simulink model "Q6"  (R2023b)
settings: Solver=VariableStepAuto  StartTime=0.0  StopTime=50  RelTol=1e-3
values from neighbouring files (symbols this model uses):
  A = [ -8.8487+(a-b)/5,           -0.0399,                     -5.55+(c+d)/10,               3.5846 ... (first row only)    [EE5101_Q1 copy.m]    (also in EE5101_Q1.m; Q3.m; Q3_reduced_order.m; Q6.m)
  B = [0.0564+b/(10+c),                       0.0319 ... (first row only)    [EE5101_Q1 copy.m]    (also in EE5101_Q1.m; Q3.m; Q3_reduced_order.m; Q6.m)
  C = [-3.2988,              -2.1932+(10*c+d)/(100+5*a),  0.037,      -0.0109 ... (first row only)    [EE5101_Q1 copy.m]    (also in EE5101_Q1.m; Q3.m; Q3_reduced_order.m; Q6.m)
settings Model: Creator=wyton  LastModifiedBy=shipingguo
settings SolverCC: AlgebraicLoopSolver=TrustRegion
settings DataIOCC: SaveState=on
settings OptimizationCC: ReuseModelBlockBuffer=off
settings DebuggingCC: UnconnectedInputMsg=warning  UnconnectedOutputMsg=warning  UnconnectedLineMsg=warning
settings ModelReferenceCC: EnableRefExpFcnMdlSchedulingChecks=on
settings RTWCC: DLArmComputeVersion=19.05

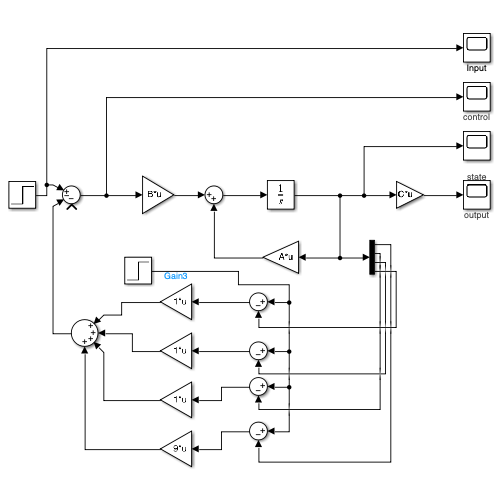
[thumbnail: Simulink's stored preview of the top-level diagram]
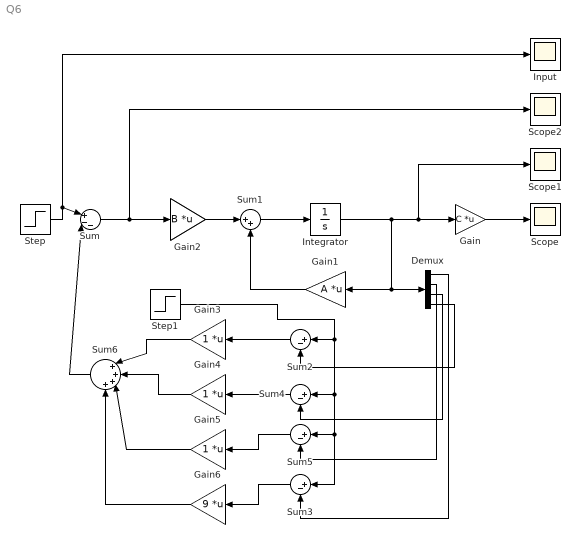
== system Q6 ==
  Demux : Demux
  Gain : Gain  Gain=C  Multiplication=Matrix(K*u)
  Gain1 : Gain  Gain=A  Multiplication=Matrix(K*u)
  Gain2 : Gain  Tag=B  Gain=B  Multiplication=Matrix(K*u)
  Gain3 : Gain  Multiplication=Matrix(K*u)
  Gain4 : Gain  Multiplication=Matrix(K*u)
  Gain5 : Gain  Multiplication=Matrix(K*u)
  Gain6 : Gain  Gain=9  Multiplication=Matrix(K*u)
  Input : Scope
  Integrator : Integrator  InitialCondition="[0.5000   -0.1000    0.1000   -0.8000]"
  Scope : Scope
      settings: AttributesFormatString=output
  Scope1 : Scope
      settings: AttributesFormatString=state
  Scope2 : Scope
      settings: AttributesFormatString=control
  Step : Step  Time=0  Before=[0,0]  After=[1,0]  SampleTime=0
  Step1 : Step  Time=0  Before=[0,0]  SampleTime=0
  Sum : Sum  Inputs=|+--
  Sum1 : Sum  Inputs=|++
  Sum{2..5} (4 alike) : Sum  Inputs=|+-
  Sum6 : Sum  Inputs=|++++
  wires:
  Step/1 -> Input/1, Sum/1
  Sum/1 -> Scope2/1, Gain2/1
  Sum1/1 -> Integrator/1
  Gain2/1 -> Sum1/1
  Integrator/1 -> Demux/1, Gain1/1, Gain/1, Scope1/1
  Gain1/1 -> Sum1/2
  Gain/1 -> Scope/1
  Step1/1 -> Sum3/1, Sum5/1, Sum4/1, Sum2/1
  Demux/4 -> Sum2/2
  Demux/3 -> Sum4/2
  Demux/2 -> Sum5/2
  Demux/1 -> Sum3/2
  Sum2/1 -> Gain3/1
  Gain3/1 -> Sum6/1
  Sum4/1 -> Gain4/1
  Sum5/1 -> Gain5/1
  Sum3/1 -> Gain6/1
  Gain5/1 -> Sum6/3
  Gain4/1 -> Sum6/2
  Gain6/1 -> Sum6/4
  Sum6/1 -> Sum/2
